simulink model "mult_lite"  (R2019b)
settings: Solver=VariableStepAuto  StartTime=0.0  StopTime=model_parameters.end  RelTol=1e-3
InitFcn:
  | [input, model_parameters] = model_multiply_init()
StartFcn:
  | [input, model_parameters] = model_multiply_init()
undefined symbols (not defined in the file or in its folder): AXI4, Lite, model_parameters
libraries: xbsIndex_r4 x5
settings Model: Creator=Ignazio  LastModifiedBy=Ignazio

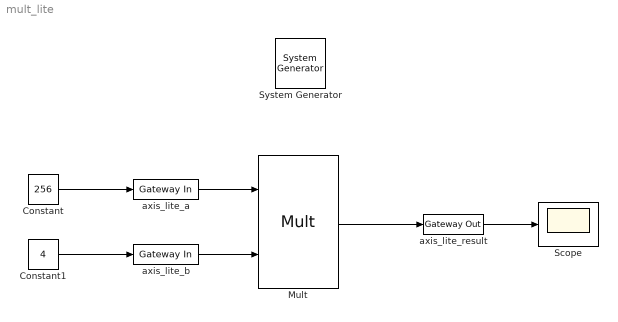
== system mult_lite ==
  " System Generator" : xbsIndex_r4/ System Generator  Tag=genX  xilinxfamily=zynquplus  part=xczu3eg  speed=-1-e  package=sbva484  synthesis_tool=Vivado  clock_wrapper=Clock Enables  directory=../IP_catalogs/mult_lite  proj_type=Vivado  Synth_file=Vivado Synthesis Defaults  Impl_file=Vivado Implementation Defaults  testbench=off  simulink_period=1/model_parameters.sampling_rate  sysclk_period=1e9/model_parameters.sampling_rate  dcm_input_clock_period=10  incr_netlist=off  trim_vbits=Everywhere in SubSystem  dbl_ovrd=According to Block Masks  core_generation=According to Block Masks  run_coregen=off  deprecated_control=off  eval_field=0  block_type=sysgen
  Constant : Constant  Value=256
  Constant1 : Constant  Value=4
  Mult : xbsIndex_r4/Mult  precision=User Defined  arith_type=Unsigned  n_bits=32  bin_pt=0  quantization=Truncate  overflow=Wrap  en=off  latency=3  use_behavioral_HDL=off  opt=Speed  use_embedded=on  optimum_pipeline=off  pipeline=on  dbl_ovrd=off  use_rpm=on  placement_style=Triangular  block_type=mult
  Scope : Scope
  axis_lite_a : xbsIndex_r4/Gateway In  gui_display_data_type=Fixed-point  arith_type=Unsigned  n_bits=32  bin_pt=0  preci_type=Single  exp_width=8  frac_width=24  rows=1  columns=1  quantization="Round  (unbiased: +/- Inf)"  overflow=Saturate  period=1/model_parameters.sampling_rate  UseAsADC=off  ADCChannel='1'  interface=AXI4-Lite  automatic_assignment=on  address_offset=hex2dec('00')  intf_name=''  intf_description=''  default_value=10  timing_constraint=None  locs_specified=off  LOCs={}  io_standard={}  inherit_from_input=off  hdl_port=on  dbl_ovrd=off  block_type=gatewayin
  axis_lite_b : xbsIndex_r4/Gateway In  gui_display_data_type=Fixed-point  arith_type=Unsigned  n_bits=32  bin_pt=0  preci_type=Single  exp_width=8  frac_width=24  rows=1  columns=1  quantization="Round  (unbiased: +/- Inf)"  overflow=Saturate  period=1/model_parameters.sampling_rate  UseAsADC=off  ADCChannel='1'  interface=AXI4-Lite  automatic_assignment=on  address_offset=hex2dec('00')  intf_name=''  intf_description=''  default_value=2  timing_constraint=None  locs_specified=off  LOCs={}  io_standard={}  inherit_from_input=off  hdl_port=on  dbl_ovrd=off  block_type=gatewayin
  axis_lite_result : xbsIndex_r4/Gateway Out  inherit_from_input=off  hdl_port=on  rows=1  columns=1  UseAsDAC=off  DACChannel='1'  interface=AXI4-Lite  automatic_assignment=on  address_offset=hex2dec('00')  intf_name=''  intf_description=''  timing_constraint=None  locs_specified=off  LOCs={}  io_standard={}  block_type=gatewayout
  wires:
  Constant/1 -> axis_lite_a/1
  axis_lite_a/1 -> Mult/1
  Constant1/1 -> axis_lite_b/1
  axis_lite_result/1 -> Scope/1
  axis_lite_b/1 -> Mult/2
  Mult/1 -> axis_lite_result/1
